simulink model "tank1"  (R2018b)
settings: Solver=ode45  StartTime=0.0  StopTime=100  RelTol=1e-3
values from neighbouring files (symbols this model uses):
  a = 0.3    [tank.m]
  A = 1    [gastank.m]    (also in tank.m = 3)
  g = 9.81    [gastank.m]    (also in tank.m)
  qzu = 5    [gastank.m]    (also in tank.m)
settings Model: Creator=Naveen  LastModifiedBy=Naveen

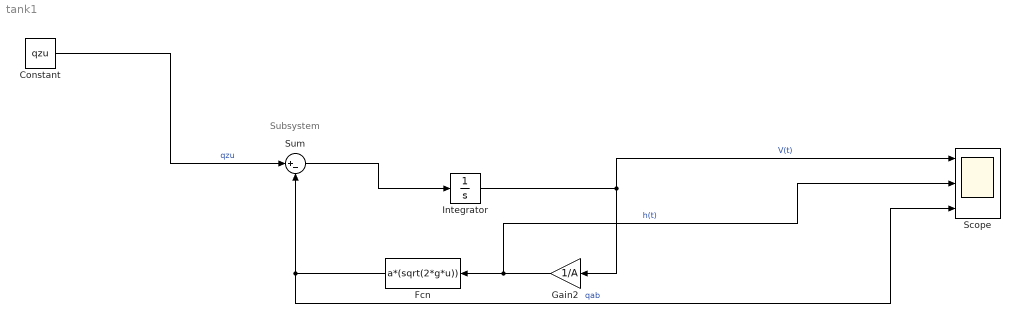
== system tank1 ==
  note: Subsystem
  Constant : Constant  Value=qzu
  Fcn : Fcn  Expr=a*(sqrt(2*g*u))
  Gain2 : Gain  Gain=1/A
  Integrator : Integrator
  Scope : Scope  NumInputPorts=3
  Sum : Sum  Inputs=|+-
  wires:
  Constant/1 -> Sum/1  "qzu"
  Integrator/1 -> Scope/1, Gain2/1  "V(t)"
  Gain2/1 -> Fcn/1, Scope/2  "h(t)"
  Fcn/1 -> Sum/2, Scope/3  "qab"
  Sum/1 -> Integrator/1
